simulink model "TP_Moteur_BO"  (R2015a)
settings: Solver=ode4  StartTime=0.0  StopTime=9999  FixedStep=Te  RelTol=1e-3
values from neighbouring files (symbols this model uses):
  Te = 0.01    [TP_Moteur_Script_Etudiant.m]
undefined symbols (not defined in the file or in its folder): EE2, K, National_Instruments, obsver, PCI
libraries: sldrtlib x2
settings Model: SimulationMode=external  Creator=sylvain  LastModifiedBy=David
settings DataIOCC: MaxDataPoints=5000  SignalLoggingSaveFormat=ModelDataLogs
settings OptimizationCC: BlockReduction=off  BooleanDataType=off  ExpressionDepthLimit=2147483647
settings DebuggingCC: SaveWithParameterizedLinksMsg=none  UnderspecifiedInitializationDetection=Classic  MergeDetectMultiDrivingBlocksExec=none  SignalResolutionControl=TryResolveAllWithWarning  MultiTaskDSMMsg=warning  MultiTaskCondExecSysMsg=none  StateNameClashWarn=warning  StrictBusMsg=None
settings HardwareCC: ProdBitPerLong=64  ProdBitPerPointer=64  ProdIntDivRoundTo=Zero  ProdEndianess=LittleEndian  ProdWordSize=64  ProdHWDeviceType=Intel->x86-64  TargetBitPerLong=64  TargetBitPerPointer=64  TargetIntDivRoundTo=Zero  TargetEndianess=LittleEndian  TargetWordSize=64  TargetHWDeviceType=Intel->x86-64
settings RTWCC: SystemTargetFile=rtwin.tlc  TemplateMakefile=rtwin.tmf  Description=Real-Time Windows Target  RTWCompilerOptimization=on
settings CodeAppCC: MaxIdLength=95
settings RTWinTargetCC: TargetPreCompLibLocation=C:\Program Files\MATLAB\MATLAB Production Server\R2015a\toolbox\sldrt\lib\win64

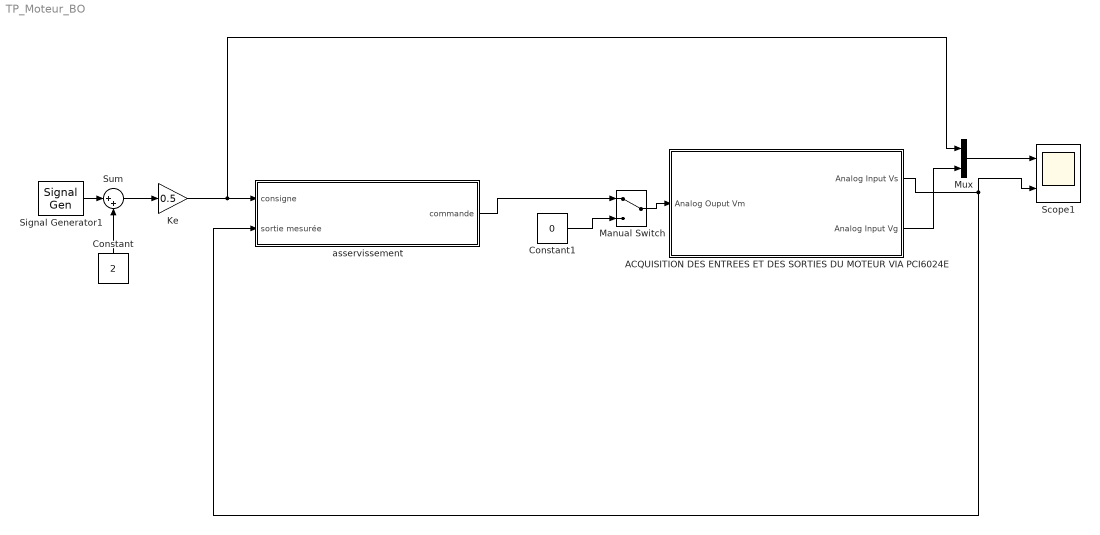
== system TP_Moteur_BO ==
  ACQUISITION DES ENTREES ET DES SORTIES DU MOTEUR VIA PCI6024E : Subsystem
  Constant : Constant  Value=2
  Constant1 : Constant  Value=0
  Ke : Gain  Gain=0.5  SaturateOnIntegerOverflow=on  OutDataTypeStr=Inherit: Same as input  ParamDataTypeStr=Inherit: Same as input
  Manual Switch : ManualSwitch
  Mux : Mux  Inputs=2
  Scope1 : Scope  NumInputPorts=2
      settings: TimeRange=3  YMin=-5.5~-5.5  YMax=5.5~5.5  SaveName=y  DataFormat=Structure
  Signal Generator1 : SignalGenerator  WaveForm=square  Amplitude=2  Frequency=0.1
  Sum : Sum  Inputs=|++  SaturateOnIntegerOverflow=on  InputSameDT=on  OutDataTypeStr=Inherit: Same as first input
  asservissement : Subsystem
  wires:
  Ke/1 -> Mux/1, asservissement/1(consigne)
  Sum/1 -> Ke/1
  Signal Generator1/1 -> Sum/1
  Constant/1 -> Sum/2
  Mux/1 -> Scope1/1
  Manual Switch/1 -> ACQUISITION DES ENTREES ET DES SORTIES DU MOTEUR VIA PCI6024E/1(Analog Ouput Vm)
  Constant1/1 -> Manual Switch/2
  ACQUISITION DES ENTREES ET DES SORTIES DU MOTEUR VIA PCI6024E/2(Analog Input Vg) -> Mux/2
  ACQUISITION DES ENTREES ET DES SORTIES DU MOTEUR VIA PCI6024E/1(Analog Input Vs) -> asservissement/2(sortie mesurée), Scope1/2
  asservissement/1(commande) -> Manual Switch/1

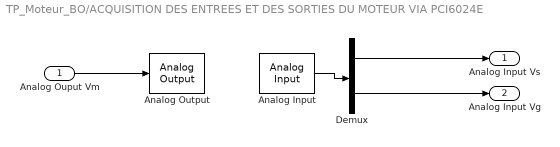
== system TP_Moteur_BO/ACQUISITION DES ENTREES ET DES SORTIES DU MOTEUR VIA PCI6024E ==
  Analog Ouput Vm : Inport
  Analog Input : sldrtlib/Analog Input  SampleTime=Te  MaxMissedTicks=10  ShowMissedTicks=off  YieldWhenWaiting=off  DrvName=National_Instruments/PCI-6024E  DrvAddress=0  DrvOptions=[0 0 0 0 0 0]  Channels=[1 2]  RangeMode=1  VoltRange=1  DataType=1
      settings: AttributesFormatString=National Instruments\nPCI-6024E [0h]
  Analog Output : sldrtlib/Analog Output  SampleTime=Te  MaxMissedTicks=10  ShowMissedTicks=off  YieldWhenWaiting=off  DrvName=National_Instruments/PCI-6024E  DrvAddress=0  DrvOptions=[0 0 0 0 0 0]  Channels=1  RangeMode=1  VoltRange=1  InitialValue=[]  FinalValue=[]
      settings: AttributesFormatString=National Instruments\nPCI-6024E [0h]
  Demux : Demux  Outputs=2
  Analog Input Vs : Outport
  Analog Input Vg : Outport  Port=2
  wires:
  Analog Input/1 -> Demux/1
  Demux/2 -> Analog Input Vg/1
  Analog Ouput Vm/1 -> Analog Output/1
  Demux/1 -> Analog Input Vs/1

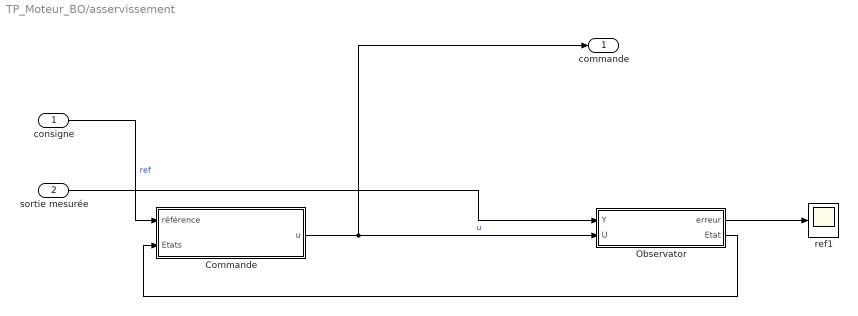
== system TP_Moteur_BO/asservissement ==
  consigne : Inport
  sortie mesurée : Inport  Port=2
  "Commande " : Subsystem
  Observator : Subsystem
  ref1 : Scope
      settings: SaveName=ScopeData4
  commande : Outport
  wires:
  consigne/1 -> "Commande "/1(référence)  "ref"
  Observator/2("Etat ") -> "Commande "/2(Etats)
  sortie mesurée/1 -> Observator/1("Y ")
  "Commande "/1(u) -> Observator/2(U), commande/1  "u"
  Observator/1(erreur) -> ref1/1

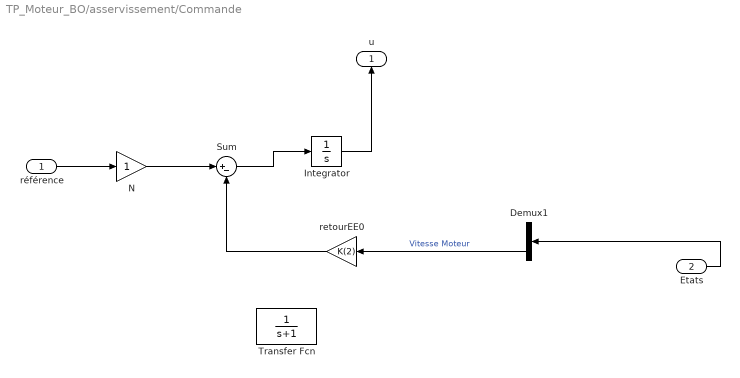
== system TP_Moteur_BO/asservissement/Commande  ==
  référence : Inport
  Etats : Inport  Port=2
  Demux1 : Demux  Outputs=2
  Integrator : Integrator
  "N " : Gain
  Sum : Sum  Inputs=|+-
  Transfer Fcn : TransferFcn  Denominator=[1 1]
  retourEE0 : Gain  Gain=K(2)
  u : Outport
  wires:
  Sum/1 -> Integrator/1
  référence/1 -> "N "/1
  Etats/1 -> Demux1/1
  retourEE0/1 -> Sum/2
  "N "/1 -> Sum/1
  Demux1/2 -> retourEE0/1  "Vitesse Moteur"
  Integrator/1 -> u/1

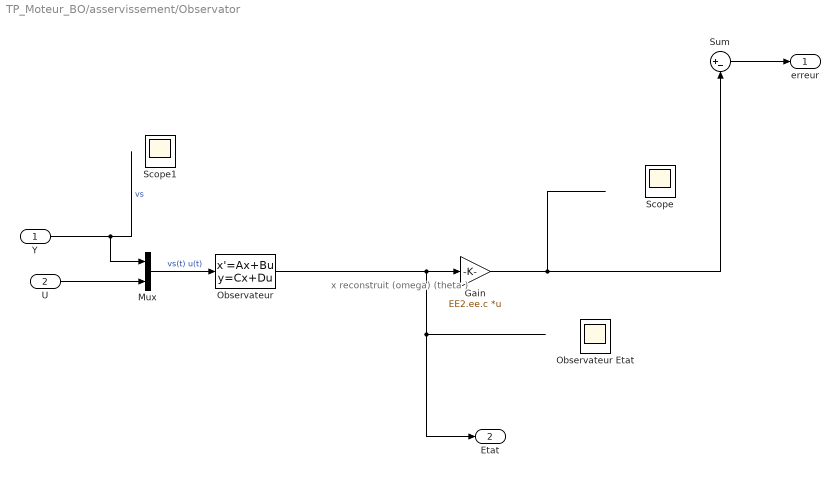
== system TP_Moteur_BO/asservissement/Observator ==
  note: x reconstruit
      | (omega)
      | (theta   )
  "Y " : Inport
  U : Inport  Port=2
  Gain : Gain  Gain=EE2.ee.c  Multiplication=Matrix(K*u)
  Mux : Mux  Inputs=2
  "Observateur " : StateSpace  A=obsver.ee.a  B=obsver.ee.b  C=obsver.ee.c  D=obsver.ee.d  X0=0
  "Observateur Etat " : Scope
  Scope : Scope
      settings: YMin=-600  YMax=600
  Scope1 : Scope
      settings: YMin=16  YMax=30  SaveName=ScopeData2
  Sum : Sum  Inputs=|+-
  erreur : Outport
  "Etat " : Outport  Port=2
  wires:
  "Observateur "/1 -> "Etat "/1, Gain/1
  "Y "/1 -> Mux/1  "vs"
  Sum/1 -> erreur/1
  Mux/1 -> "Observateur "/1  "vs(t) u(t)"
  Gain/1 -> Sum/2
  U/1 -> Mux/2
